simulink model "Practica6_ControladorOptimo"  (R2022a)
settings: Solver=ode4  StartTime=0.0  StopTime=15  FixedStep=0.001  RelTol=1e-3
model workspace (MAT data in the model file):
  ci = 5
undefined symbols (not defined in the file or in its folder): K
settings Model: Creator=edgar  LastModifiedBy=Anahi Monserrat
settings ModelReferenceCC: EnableRefExpFcnMdlSchedulingChecks=off
settings RTWCC: Description=Generic Real-Time Target

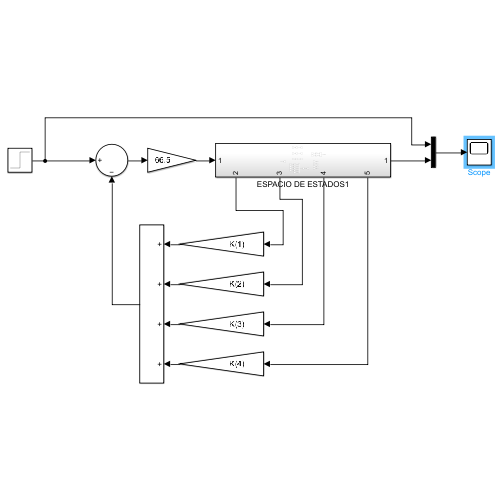
[thumbnail: Simulink's stored preview of the top-level diagram]
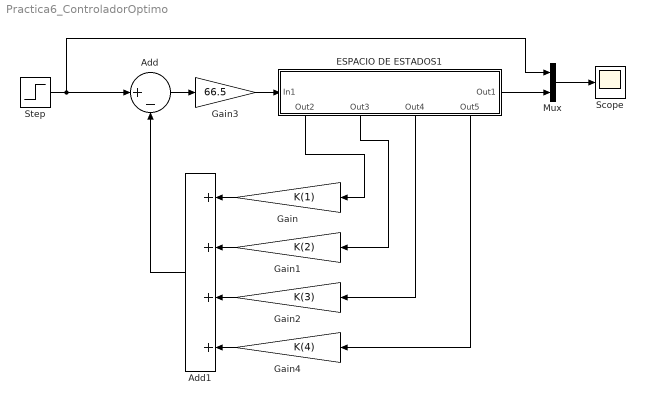
== system Practica6_ControladorOptimo ==
  Add : Sum  Inputs=|+-
  Add1 : Sum  Inputs=++++
  ESPACIO DE ESTADOS1 : Subsystem
      settings: PortSchema="{\"entries\":[{\"content\":{\"sides\":[{\"content\":{\"connectorIds\":[\"In1\"]},\"type\":\"ConnectorPlacement.EquallySpacedRectSide\",\"uuid\":\"e4c7e91e-e27a-4516-8912-0ffb8324b1cf\"},{\"content\":{\"connectorIds\":[\"Out1\"],\"side\":\"RIGHT\"},\"type\":\"ConnectorPlacement.EquallySpacedRectSide\",\"uuid\":\"c8b6f25f-762c-42f8-84b8-6d4e17a9e409\"},{\"content\":{\"connectorIds\":[],\"side\":\"TOP\"},\"type\":\"ConnectorPlacement.EquallySpacedRectSide\",\"uuid\":\"20a6fbcd-96ab-4412-bae7-78daeec6f97a\"},{\"content\":{\"connectorIds\":[\"Out2\",\"Out3\",\"Out4\",\"Out5\"],\"side\":\"BOTTOM\"},\"type\":\"ConnectorPlacement.EquallySpacedRectSide\",\"uuid\":\"214e34fb-e27d-4adf-9fcb-27d6061738d6\"}]},\"type\":\"ConnectorPlacement.EquallySpacedConnector\",\"uuid\":\"46eb5afa-d204-4a9b-9a44-848bb687e783\"}],\"packageUris\":[\"http://schema.mathworks.com/mf0/Connector/R2020b\"],\"version\":\"1.0\"}"
  Gain : Gain  Gain=K(1)
  Gain1 : Gain  Gain=K(2)
  Gain2 : Gain  Gain=K(3)
  Gain3 : Gain  Gain=66.5
  Gain4 : Gain  Gain=K(4)
  Mux : Mux  Inputs=2
  Scope : Scope
  Step : Step  SampleTime=0
  wires:
  Gain1/1 -> Add1/2
  ESPACIO DE ESTADOS1/1(Out1) -> Mux/2
  Gain2/1 -> Add1/3
  Mux/1 -> Scope/1
  Gain4/1 -> Add1/4
  Add1/1 -> Add/2
  Gain/1 -> Add1/1
  Add/1 -> Gain3/1
  ESPACIO DE ESTADOS1/2(Out2) -> Gain/1
  ESPACIO DE ESTADOS1/3(Out3) -> Gain1/1
  ESPACIO DE ESTADOS1/4(Out4) -> Gain2/1
  ESPACIO DE ESTADOS1/5(Out5) -> Gain4/1
  Step/1 -> Add/1, Mux/1
  Gain3/1 -> ESPACIO DE ESTADOS1/1(In1)

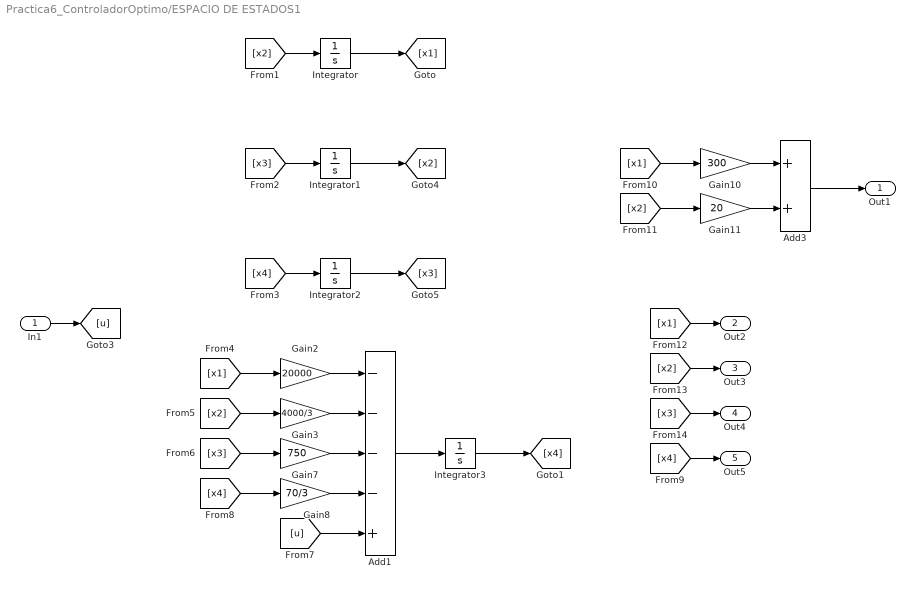
== system Practica6_ControladorOptimo/ESPACIO DE ESTADOS1 ==
  In1 : Inport
  Add1 : Sum  Inputs=----+
  Add3 : Sum
  Gain10 : Gain  Gain=300
  Gain11 : Gain  Gain=20
  Gain2 : Gain  Gain=20000
  Gain3 : Gain  Gain=4000/3
  Gain7 : Gain  Gain=750
  Gain8 : Gain  Gain=70/3
  Integrator{,1..3} (4 alike) : Integrator
  Out1 : Outport
  Out2 : Outport  Port=2
  Out3 : Outport  Port=3
  Out4 : Outport  Port=4
  Out5 : Outport  Port=5
  wires:
  [x1] -> Out2/1
  [x2] -> Out3/1
  [x3] -> Out4/1
  [x1] -> Gain10/1
  Gain10/1 -> Add3/1
  Gain11/1 -> Add3/2
  In1/1 -> [u]
  [x2] -> Gain11/1
  Add3/1 -> Out1/1
  [x4] -> Out5/1
  [x4] -> Integrator2/1
  [x3] -> Integrator1/1
  Integrator/1 -> [x1]
  [x2] -> Integrator/1
  Add1/1 -> Integrator3/1
  Integrator3/1 -> [x4]
  [x2] -> Gain3/1
  [x1] -> Gain2/1
  Gain3/1 -> Add1/2
  [x4] -> Gain8/1
  Gain8/1 -> Add1/4
  [u] -> Add1/5
  Integrator1/1 -> [x2]
  [x3] -> Gain7/1
  Gain2/1 -> Add1/1
  Gain7/1 -> Add1/3
  Integrator2/1 -> [x3]
